simulink model "feed"  (R2025a)
settings: Solver=FixedStepAuto  StartTime=0.0  StopTime=0.1  FixedStep=1e-5  RelTol=1e-3
values from neighbouring files (symbols this model uses):
  Ki = 20    [control_5_test.m]    (also in feed_forward.m = 100)
  Kp = 20    [control_5_test.m]    (also in feed_forward.m = 0.707)
  wn = 2*pi*350    (= 2199.11485751)    [feed_forward.m]
  zeta = 0.707    [feed_forward.m]
settings Model: Creator=moon  LastModifiedBy=moon

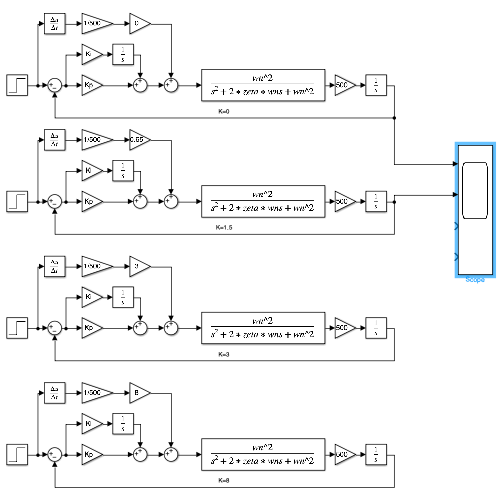
[thumbnail: Simulink's stored preview of the top-level diagram]
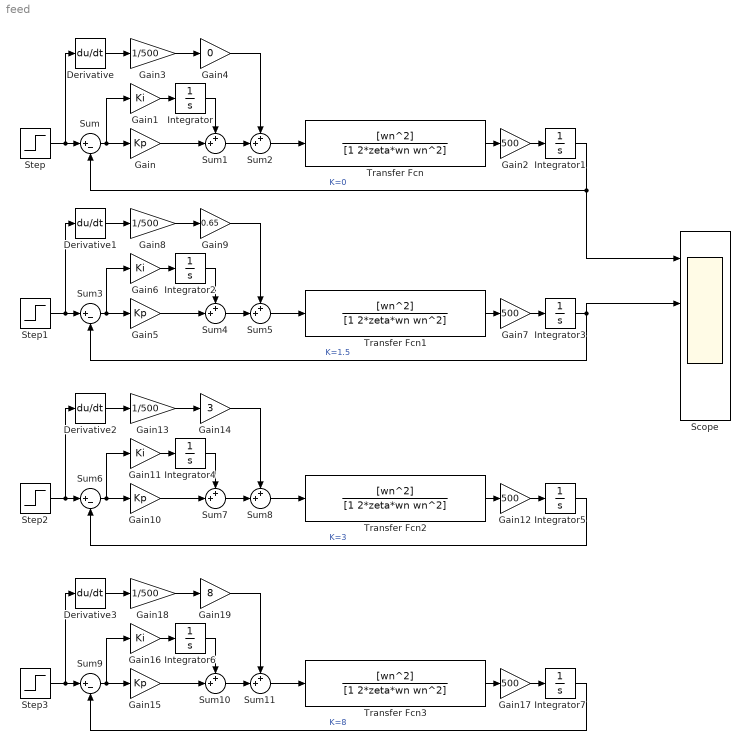
== system feed ==
  Derivative{,1..3} (4 alike) : Derivative
  Gain{,5,10,15} (4 alike) : Gain  Gain=Kp
  Gain{1,6,11,16} (4 alike) : Gain  Gain=Ki
  Gain{2,7,12,17} (4 alike) : Gain  Gain=500
  Gain{3,8,13,18} (4 alike) : Gain  Gain=1/500
  Gain14 : Gain  Gain=3
  Gain19 : Gain  Gain=8
  Gain4 : Gain  Gain=0
  Gain9 : Gain  Gain=0.65
  Integrator{,1..7} (8 alike) : Integrator
  Scope : Scope  NumInputPorts=4
      settings: ActiveDisplayYMinimum=-0.15418462191281521  ActiveDisplayYMaximum=1.3876615972153372
  Step{,1..3} (4 alike) : Step  Time=0.02  SampleTime=0
  Sum{,3,6,9} (4 alike) : Sum  Inputs=|+-
  Sum{1..2,4..5,7..8,10..11} (8 alike) : Sum  Inputs=++|
  Transfer Fcn{,1..3} (4 alike) : TransferFcn  Numerator=[wn^2]  Denominator=[1 2*zeta*wn wn^2]
  wires:
  Step/1 -> Derivative/1, Sum/1
  Sum/1 -> Gain1/1, Gain/1
  Gain1/1 -> Integrator/1
  Integrator/1 -> Sum1/1
  Gain/1 -> Sum1/2
  Sum1/1 -> Sum2/2
  Sum2/1 -> Transfer Fcn/1
  Transfer Fcn/1 -> Gain2/1
  Gain2/1 -> Integrator1/1
  Integrator1/1 -> Scope/1, Sum/2  "K=0"
  Derivative/1 -> Gain3/1
  Gain3/1 -> Gain4/1
  Gain4/1 -> Sum2/1
  Gain7/1 -> Integrator3/1
  Sum3/1 -> Gain6/1, Gain5/1
  Integrator2/1 -> Sum4/1
  Gain8/1 -> Gain9/1
  Derivative1/1 -> Gain8/1
  Sum5/1 -> Transfer Fcn1/1
  Step1/1 -> Derivative1/1, Sum3/1
  Transfer Fcn1/1 -> Gain7/1
  Gain5/1 -> Sum4/2
  Integrator3/1 -> Sum3/2, Scope/2  "K=1.5"
  Sum4/1 -> Sum5/2
  Gain6/1 -> Integrator2/1
  Gain9/1 -> Sum5/1
  Gain12/1 -> Integrator5/1
  Sum6/1 -> Gain11/1, Gain10/1
  Integrator4/1 -> Sum7/1
  Gain13/1 -> Gain14/1
  Derivative2/1 -> Gain13/1
  Sum8/1 -> Transfer Fcn2/1
  Step2/1 -> Derivative2/1, Sum6/1
  Transfer Fcn2/1 -> Gain12/1
  Gain10/1 -> Sum7/2
  Integrator5/1 -> Sum6/2  "K=3"
  Sum7/1 -> Sum8/2
  Gain11/1 -> Integrator4/1
  Gain14/1 -> Sum8/1
  Gain17/1 -> Integrator7/1
  Sum9/1 -> Gain16/1, Gain15/1
  Integrator6/1 -> Sum10/1
  Gain18/1 -> Gain19/1
  Derivative3/1 -> Gain18/1
  Sum11/1 -> Transfer Fcn3/1
  Step3/1 -> Derivative3/1, Sum9/1
  Transfer Fcn3/1 -> Gain17/1
  Gain15/1 -> Sum10/2
  Integrator7/1 -> Sum9/2  "K=8"
  Sum10/1 -> Sum11/2
  Gain16/1 -> Integrator6/1
  Gain19/1 -> Sum11/1
